simulink model "Lab3_Part1_Q4"  (R2020a)
settings: Solver=VariableStepAuto  StartTime=0.0  StopTime=10.0  RelTol=1e-3
libraries: commchan3 x1, commrandsrc3 x1, commsink2 x1, dspsigops x1
settings Model: Creator=pyrpo  LastModifiedBy=pyrpo

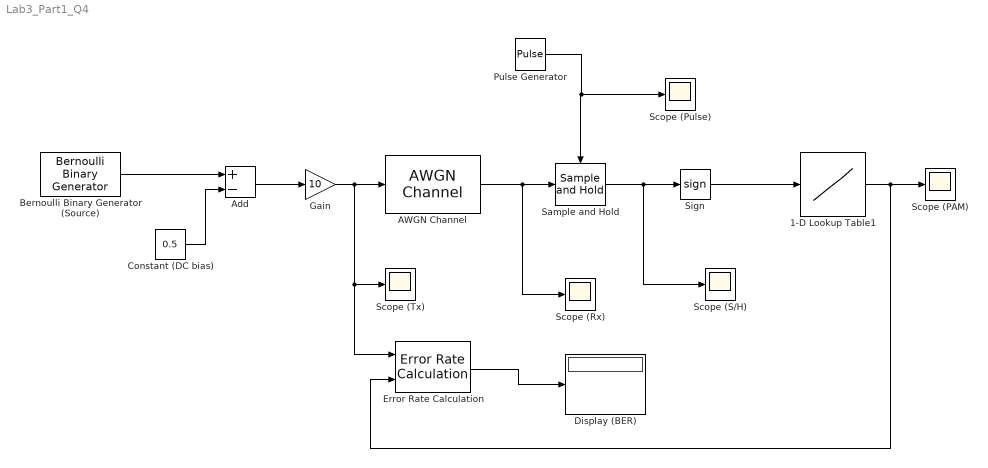
== system Lab3_Part1_Q4 ==
  1-D Lookup Table1 : Lookup_n-D  NumberOfTableDimensions=1  LookupTableObject=''  BreakpointsForDimension1=[-1,0,1]  BreakpointsForDimension1FirstPoint=10  BreakpointsForDimension2FirstPoint=10  BreakpointsForDimension1Spacing=12  BreakpointsForDimension2Spacing=12  IndexSearchMethod=Evenly spaced points  Table=[-5,-5,5]  InterpMethod=Flat  DiagnosticForOutOfRangeInput=Error  InternalRulePriority=Speed  RndMeth=Simplest  InputSameDT=on
  AWGN Channel : commchan3/AWGN Channel  InputProcessing=Columns as channels (frame based)  seed=67  noiseMode="Signal to noise ratio  (Eb/No)"  EbNodB=10  EsNodB=10  SNRdB=10  bitsPerSym=1  Ps=25  Tsym=1e-3  variance=1
  Add : Sum  Inputs=+-
  Bernoulli Binary Generator (Source) : commrandsrc3/Bernoulli Binary Generator  ProbabilityOfZero=0.5  SeedSource=Auto  Seed=0  SampleTime=1e-3  SamplesPerFrame=1  OutputDataType=double  SimulateUsing=Interpreted execution
  Constant (DC bias) : Constant  Value=0.5
  Display (BER) : Display
  Error Rate Calculation : commsink2/Error Rate Calculation  N=1  st_delay=0  cp_mode=Entire frame  subframe=[]  PMode=Port  WsName=ErrorVec  RsMode2=off  stop=on  numErr=200  maxBits=1e6
  Gain : Gain  Gain=10
  Pulse Generator : DiscretePulseGenerator  PhaseDelay=1  SampleTime=0.5e-3
  Sample and Hold : dspsigops/Sample and Hold  trig=Rising edge  initCond=0  latchinput=off
  Scope (PAM) : Scope
  Scope (Pulse) : Scope
  Scope (Rx) : Scope
  Scope (S/H) : Scope
  Scope (Tx) : Scope
  Sign : Signum
  wires:
  Bernoulli Binary Generator (Source)/1 -> Add/1
  Constant (DC bias)/1 -> Add/2
  Add/1 -> Gain/1
  AWGN Channel/1 -> Scope (Rx)/1, Sample and Hold/1
  Sample and Hold/1 -> Scope (S/H)/1, Sign/1
  1-D Lookup Table1/1 -> Error Rate Calculation/2, Scope (PAM)/1
  Pulse Generator/1 -> Scope (Pulse)/1, Sample and Hold/Trigger
  Gain/1 -> Scope (Tx)/1, Error Rate Calculation/1, AWGN Channel/1
  Error Rate Calculation/1 -> Display (BER)/1
  Sign/1 -> 1-D Lookup Table1/1
